simulink model "tutorial14_foc"  (R2025a)
settings: Solver=VariableStepAuto  StartTime=0.0  StopTime=0.15  RelTol=1e-3
settings Model: Creator=xing2  LastModifiedBy=xing2

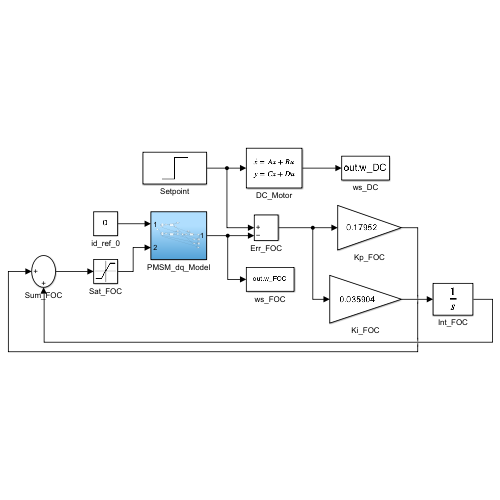
[thumbnail: Simulink's stored preview of the top-level diagram]
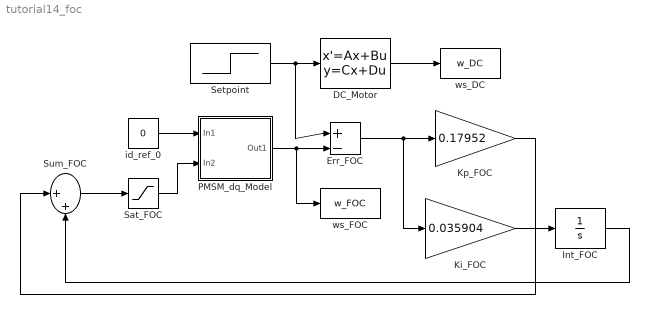
== system tutorial14_foc ==
  DC_Motor : StateSpace  A=[-1000 -7.5;30 -0.02]  B=[500;0]  C=[0 1]  D=0  InitialCondition=[0; 0]
  Err_FOC : Sum  Inputs=|+-
  Int_FOC : Integrator
  Ki_FOC : Gain  Gain=0.035904
  Kp_FOC : Gain  Gain=0.17952
  PMSM_dq_Model : Subsystem
  Sat_FOC : Saturate  UpperLimit=24  LowerLimit=-24
  Setpoint : Step  Time=0.01  After=200  SampleTime=0
  Sum_FOC : Sum  Inputs=|++
  id_ref_0 : Constant  Value=0
  ws_DC : ToWorkspace  VariableName=w_DC  SaveFormat=Timeseries  SampleTime=-1
  ws_FOC : ToWorkspace  VariableName=w_FOC  SaveFormat=Timeseries  SampleTime=-1
  wires:
  DC_Motor/1 -> ws_DC/1
  Sum_FOC/1 -> Sat_FOC/1
  id_ref_0/1 -> PMSM_dq_Model/1(In1)
  Int_FOC/1 -> Sum_FOC/2
  Sat_FOC/1 -> PMSM_dq_Model/2(In2)
  Setpoint/1 -> DC_Motor/1, Err_FOC/1
  Err_FOC/1 -> Ki_FOC/1, Kp_FOC/1
  PMSM_dq_Model/1(Out1) -> Err_FOC/2, ws_FOC/1
  Kp_FOC/1 -> Sum_FOC/1
  Ki_FOC/1 -> Int_FOC/1

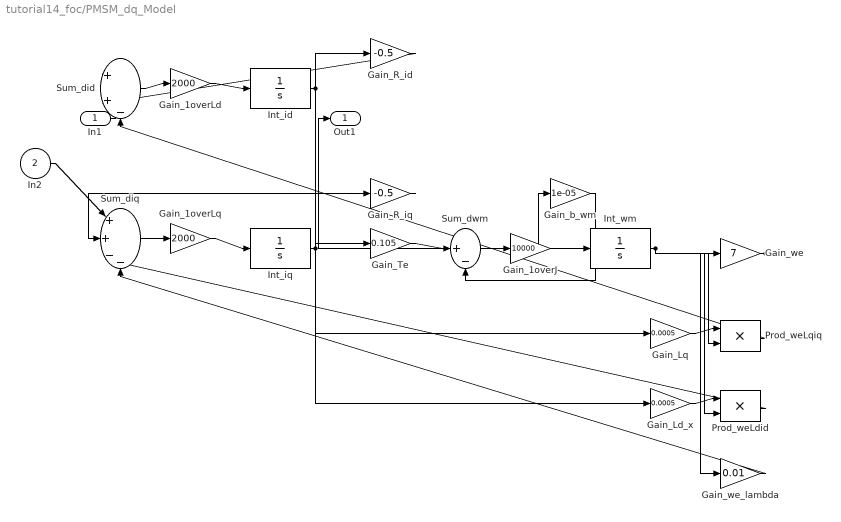
== system tutorial14_foc/PMSM_dq_Model ==
  In1 : Inport
  In2 : Inport  Port=2
  Gain_1overJ : Gain  Gain=10000
  Gain_1overLd : Gain  Gain=2000
  Gain_1overLq : Gain  Gain=2000
  Gain_Ld_x : Gain  Gain=0.0005
  Gain_Lq : Gain  Gain=0.0005
  Gain_R_id : Gain  Gain=-0.5
  Gain_R_iq : Gain  Gain=-0.5
  Gain_Te : Gain  Gain=0.105
  Gain_b_wm : Gain  Gain=1e-05
  Gain_we : Gain  Gain=7
  Gain_we_lambda : Gain  Gain=0.01
  Int_id : Integrator
  Int_iq : Integrator
  Int_wm : Integrator
  Prod_weLdid : Product  Inputs=**
  Prod_weLqiq : Product  Inputs=**
  Sum_did : Sum  Inputs=|++-
  Sum_diq : Sum  Inputs=|++--
  Sum_dwm : Sum  Inputs=|+-
  Out1 : Outport
  wires:
  In1/1 -> Sum_did/1
  Gain_R_id/1 -> Sum_did/2
  Sum_did/1 -> Gain_1overLd/1
  Gain_1overLd/1 -> Int_id/1
  In2/1 -> Sum_diq/1
  Gain_R_iq/1 -> Sum_diq/2
  Sum_diq/1 -> Gain_1overLq/1
  Gain_1overLq/1 -> Int_iq/1
  Int_iq/1 -> Gain_Te/1, Gain_Lq/1, Gain_R_iq/1
  Gain_Te/1 -> Sum_dwm/1
  Gain_b_wm/1 -> Sum_dwm/2
  Sum_dwm/1 -> Gain_1overJ/1
  Gain_1overJ/1 -> Int_wm/1
  Int_wm/1 -> Gain_we/1, Gain_b_wm/1, Out1/1
  Gain_Lq/1 -> Prod_weLqiq/1
  Gain_we/1 -> Prod_weLqiq/2, Prod_weLdid/2, Gain_we_lambda/1
  Int_id/1 -> Gain_Ld_x/1, Gain_R_id/1
  Gain_Ld_x/1 -> Prod_weLdid/1
  Prod_weLqiq/1 -> Sum_did/3
  Prod_weLdid/1 -> Sum_diq/3
  Gain_we_lambda/1 -> Sum_diq/4
